simulink model "DFADAS2_SenFus_v1_201204RC_training_210115"  (R2018b)
settings: Solver=FixedStepDiscrete  StartTime=0.0  StopTime=inf  FixedStep=0.002  RelTol=1e-3  EnableMultiTasking=on
PreLoadFcn:
  | RTWConfigurationCB('preloadfcn', bdroot);
libraries: canmsglib x108, simulink x48, canfdmsglib x12
(part 8 of 28)

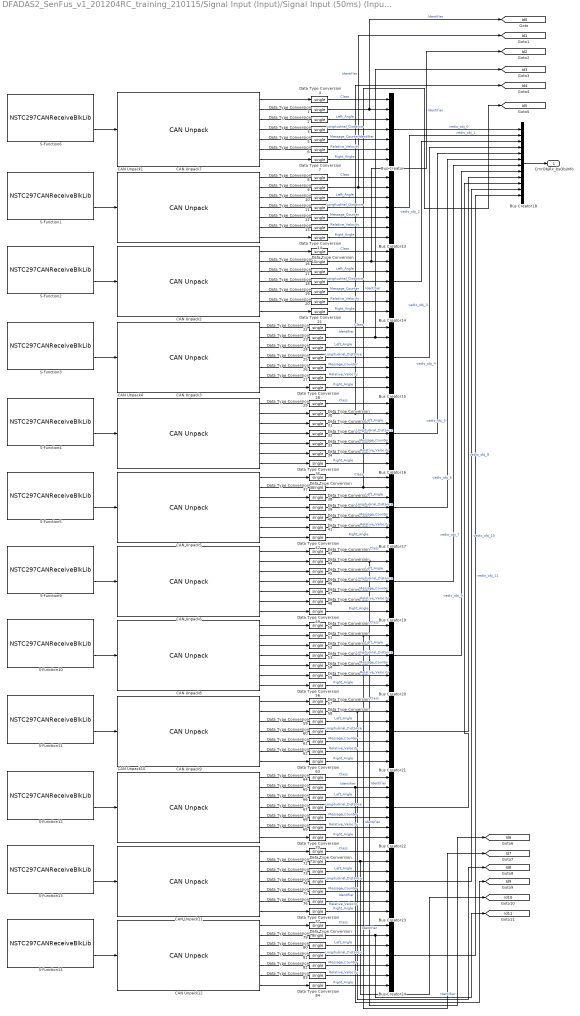
== system DFADAS2_SenFus_v1_201204RC_training_210115/Signal Input (Input)/Signal Input (50ms) (Input50)/Cmr/Camera Objects Information (CmrObjInfo) ==
  Bus Creator{,13..17,19..24} (12 alike) : BusCreator  Inputs=7
  Bus Creator18 : BusCreator  Inputs=12
  CAN Unpack1 : canmsglib/CAN Unpack  CANdbFile=F:\V_control\ADAS ECU-Sensor CAN_V2_20190314(1).dbc  MsgList=Video_Object_1_A  MsgName=Video_Object_1_A  MsgIDType=Standard (11-bit identifier)  MsgIdentifier=1796  MsgLength=8  SignalInfo=Class_704$56$3$2$2$1$0$1$0$0$7$#Identifier_704$1$7$2$2$1$0$1$0$0$127$#Left_Angle_704$41$13$2$1$1$0$2.000000e-04$0$-8.192000e-01$8.190000e-01$#Longitudinal_Distance_704$20$12$2$2$1$0$5.000000e-02$0$0$2.047500e+02$#Message_Counter_704$38$2$2$2$1$0$1$0$0$3$#Relative_Velocity_704$24$12$2$1$1$0$5.000000e-02$0$-1.024000e+02$1.023500e+02$#Right_Angle_704$59$13$2$1$1$0$2.000000e-04$0$-8.192000e-01$8.190000e-01$#  NSignals=7  IDPort=off  TimestampPort=off  ErrorPort=off  RemotePort=off  LengthPort=off  StatusPort=off  StartBits=str2num('[int32(56);int32(1);int32(41);int32(20);int32(38);int32(24);int32(59)]')  SignalSizes=str2num('[int32(3);int32(7);int32(13);int32(12);int32(2);int32(12);int32(13)]')  ByteOrders=str2num('[int32(2);int32(2);int32(2);int32(2);int32(2);int32(2);int32(2)]')  DataTypes=str2num('[int32(2);int32(2);int32(1);int32(2);int32(2);int32(1);int32(1)]')  MultiplexTypes=str2num('[int32(1);int32(1);int32(1);int32(1);int32(1);int32(1);int32(1)]')  MultiplexValues=str2num('[double(0);double(0);double(0);double(0);double(0);double(0);double(0)]')  Factors=str2num('[double(1);double(1);double(2.000000e-04);double(5.000000e-02);double(1);double(5.000000e-02);double(2.000000e-04)]')  Offsets=str2num('[double(0);double(0);double(0);double(0);double(0);double(0);double(0)]')  Minimums=str2num('[double(0);double(0);double(-8.192000e-01);double(0);double(0);double(-1.024000e+02);double(-8.192000e-01)]')  Maximums=str2num('[double(7);double(127);double(8.190000e-01);double(2.047500e+02);double(3);double(1.023500e+02);double(8.190000e-01)]')  ApplyMinMax=off
      settings: SourceProductName=Simulink Real-Time  SourceProductBaseCode=XP  DataFormat=CANdb specified signals
  CAN Unpack10 : canmsglib/CAN Unpack  CANdbFile=F:\V_control\ADAS ECU-Sensor CAN_V2_20190314(1).dbc  MsgList=Video_Object_9_A  MsgName=Video_Object_9_A  MsgIDType=Standard (11-bit identifier)  MsgIdentifier=1828  MsgLength=8  SignalInfo=Class_724$56$3$2$2$1$0$1$0$0$7$#Identifier_724$1$7$2$2$1$0$1$0$0$127$#Left_Angle_724$41$13$2$1$1$0$2.000000e-04$0$-8.192000e-01$8.190000e-01$#Longitudinal_Distance_724$20$12$2$2$1$0$5.000000e-02$0$0$2.047500e+02$#Message_Counter_724$38$2$2$2$1$0$1$0$0$3$#Relative_Velocity_724$24$12$2$1$1$0$5.000000e-02$0$-1.024000e+02$1.023500e+02$#Right_Angle_724$59$13$2$1$1$0$2.000000e-04$0$-8.192000e-01$8.190000e-01$#  NSignals=7  IDPort=off  TimestampPort=off  ErrorPort=off  RemotePort=off  LengthPort=off  StatusPort=off  StartBits=str2num('[int32(56);int32(1);int32(41);int32(20);int32(38);int32(24);int32(59)]')  SignalSizes=str2num('[int32(3);int32(7);int32(13);int32(12);int32(2);int32(12);int32(13)]')  ByteOrders=str2num('[int32(2);int32(2);int32(2);int32(2);int32(2);int32(2);int32(2)]')  DataTypes=str2num('[int32(2);int32(2);int32(1);int32(2);int32(2);int32(1);int32(1)]')  MultiplexTypes=str2num('[int32(1);int32(1);int32(1);int32(1);int32(1);int32(1);int32(1)]')  MultiplexValues=str2num('[double(0);double(0);double(0);double(0);double(0);double(0);double(0)]')  Factors=str2num('[double(1);double(1);double(2.000000e-04);double(5.000000e-02);double(1);double(5.000000e-02);double(2.000000e-04)]')  Offsets=str2num('[double(0);double(0);double(0);double(0);double(0);double(0);double(0)]')  Minimums=str2num('[double(0);double(0);double(-8.192000e-01);double(0);double(0);double(-1.024000e+02);double(-8.192000e-01)]')  Maximums=str2num('[double(7);double(127);double(8.190000e-01);double(2.047500e+02);double(3);double(1.023500e+02);double(8.190000e-01)]')  ApplyMinMax=off
      settings: SourceProductName=Simulink Real-Time  SourceProductBaseCode=XP  DataFormat=CANdb specified signals
  CAN Unpack11 : canmsglib/CAN Unpack  CANdbFile=F:\V_control\ADAS ECU-Sensor CAN_V2_20190314(1).dbc  MsgList=Video_Object_10_A  MsgName=Video_Object_10_A  MsgIDType=Standard (11-bit identifier)  MsgIdentifier=1832  MsgLength=8  SignalInfo=Class_728$56$3$2$2$1$0$1$0$0$7$#Identifier_728$1$7$2$2$1$0$1$0$0$127$#Left_Angle_728$41$13$2$1$1$0$2.000000e-04$0$-8.192000e-01$8.190000e-01$#Longitudinal_Distance_728$20$12$2$2$1$0$5.000000e-02$0$0$2.047500e+02$#Message_Counter_728$38$2$2$2$1$0$1$0$0$3$#Relative_Velocity_728$24$12$2$1$1$0$5.000000e-02$0$-1.024000e+02$1.023500e+02$#Right_Angle_728$59$13$2$1$1$0$2.000000e-04$0$-8.192000e-01$8.190000e-01$#  NSignals=7  IDPort=off  TimestampPort=off  ErrorPort=off  RemotePort=off  LengthPort=off  StatusPort=off  StartBits=str2num('[int32(56);int32(1);int32(41);int32(20);int32(38);int32(24);int32(59)]')  SignalSizes=str2num('[int32(3);int32(7);int32(13);int32(12);int32(2);int32(12);int32(13)]')  ByteOrders=str2num('[int32(2);int32(2);int32(2);int32(2);int32(2);int32(2);int32(2)]')  DataTypes=str2num('[int32(2);int32(2);int32(1);int32(2);int32(2);int32(1);int32(1)]')  MultiplexTypes=str2num('[int32(1);int32(1);int32(1);int32(1);int32(1);int32(1);int32(1)]')  MultiplexValues=str2num('[double(0);double(0);double(0);double(0);double(0);double(0);double(0)]')  Factors=str2num('[double(1);double(1);double(2.000000e-04);double(5.000000e-02);double(1);double(5.000000e-02);double(2.000000e-04)]')  Offsets=str2num('[double(0);double(0);double(0);double(0);double(0);double(0);double(0)]')  Minimums=str2num('[double(0);double(0);double(-8.192000e-01);double(0);double(0);double(-1.024000e+02);double(-8.192000e-01)]')  Maximums=str2num('[double(7);double(127);double(8.190000e-01);double(2.047500e+02);double(3);double(1.023500e+02);double(8.190000e-01)]')  ApplyMinMax=off
      settings: SourceProductName=Simulink Real-Time  SourceProductBaseCode=XP  DataFormat=CANdb specified signals
  CAN Unpack12 : canmsglib/CAN Unpack  CANdbFile=F:\V_control\ADAS ECU-Sensor CAN_V2_20190314(1).dbc  MsgList=Video_Object_11_A  MsgName=Video_Object_11_A  MsgIDType=Standard (11-bit identifier)  MsgIdentifier=1836  MsgLength=8  SignalInfo=Class_72C$56$3$2$2$1$0$1$0$0$7$#Identifier_72C$1$7$2$2$1$0$1$0$0$127$#Left_Angle_72C$41$13$2$1$1$0$2.000000e-04$0$-8.192000e-01$8.190000e-01$#Longitudinal_Distance_72C$20$12$2$2$1$0$5.000000e-02$0$0$2.047500e+02$#Message_Counter_72C$38$2$2$2$1$0$1$0$0$3$#Relative_Velocity_72C$24$12$2$1$1$0$5.000000e-02$0$-1.024000e+02$1.023500e+02$#Right_Angle_72C$59$13$2$1$1$0$2.000000e-04$0$-8.192000e-01$8.190000e-01$#  NSignals=7  IDPort=off  TimestampPort=off  ErrorPort=off  RemotePort=off  LengthPort=off  StatusPort=off  StartBits=str2num('[int32(56);int32(1);int32(41);int32(20);int32(38);int32(24);int32(59)]')  SignalSizes=str2num('[int32(3);int32(7);int32(13);int32(12);int32(2);int32(12);int32(13)]')  ByteOrders=str2num('[int32(2);int32(2);int32(2);int32(2);int32(2);int32(2);int32(2)]')  DataTypes=str2num('[int32(2);int32(2);int32(1);int32(2);int32(2);int32(1);int32(1)]')  MultiplexTypes=str2num('[int32(1);int32(1);int32(1);int32(1);int32(1);int32(1);int32(1)]')  MultiplexValues=str2num('[double(0);double(0);double(0);double(0);double(0);double(0);double(0)]')  Factors=str2num('[double(1);double(1);double(2.000000e-04);double(5.000000e-02);double(1);double(5.000000e-02);double(2.000000e-04)]')  Offsets=str2num('[double(0);double(0);double(0);double(0);double(0);double(0);double(0)]')  Minimums=str2num('[double(0);double(0);double(-8.192000e-01);double(0);double(0);double(-1.024000e+02);double(-8.192000e-01)]')  Maximums=str2num('[double(7);double(127);double(8.190000e-01);double(2.047500e+02);double(3);double(1.023500e+02);double(8.190000e-01)]')  ApplyMinMax=off
      settings: SourceProductName=Simulink Real-Time  SourceProductBaseCode=XP  DataFormat=CANdb specified signals
  CAN Unpack2 : canmsglib/CAN Unpack  CANdbFile=F:\V_control\ADAS ECU-Sensor CAN_V2_20190314(1).dbc  MsgList=Video_Object_2_A  MsgName=Video_Object_2_A  MsgIDType=Standard (11-bit identifier)  MsgIdentifier=1800  MsgLength=8  SignalInfo=Class_708$56$3$2$2$1$0$1$0$0$7$#Identifier_708$1$7$2$2$1$0$1$0$0$127$#Left_Angle_708$41$13$2$1$1$0$2.000000e-04$0$-8.192000e-01$8.190000e-01$#Longitudinal_Distance_708$20$12$2$2$1$0$5.000000e-02$0$0$2.047500e+02$#Message_Counter_708$38$2$2$2$1$0$1$0$0$3$#Relative_Velocity_708$24$12$2$1$1$0$5.000000e-02$0$-1.024000e+02$1.023500e+02$#Right_Angle_708$59$13$2$1$1$0$2.000000e-04$0$-8.192000e-01$8.190000e-01$#  NSignals=7  IDPort=off  TimestampPort=off  ErrorPort=off  RemotePort=off  LengthPort=off  StatusPort=off  StartBits=str2num('[int32(56);int32(1);int32(41);int32(20);int32(38);int32(24);int32(59)]')  SignalSizes=str2num('[int32(3);int32(7);int32(13);int32(12);int32(2);int32(12);int32(13)]')  ByteOrders=str2num('[int32(2);int32(2);int32(2);int32(2);int32(2);int32(2);int32(2)]')  DataTypes=str2num('[int32(2);int32(2);int32(1);int32(2);int32(2);int32(1);int32(1)]')  MultiplexTypes=str2num('[int32(1);int32(1);int32(1);int32(1);int32(1);int32(1);int32(1)]')  MultiplexValues=str2num('[double(0);double(0);double(0);double(0);double(0);double(0);double(0)]')  Factors=str2num('[double(1);double(1);double(2.000000e-04);double(5.000000e-02);double(1);double(5.000000e-02);double(2.000000e-04)]')  Offsets=str2num('[double(0);double(0);double(0);double(0);double(0);double(0);double(0)]')  Minimums=str2num('[double(0);double(0);double(-8.192000e-01);double(0);double(0);double(-1.024000e+02);double(-8.192000e-01)]')  Maximums=str2num('[double(7);double(127);double(8.190000e-01);double(2.047500e+02);double(3);double(1.023500e+02);double(8.190000e-01)]')  ApplyMinMax=off
      settings: SourceProductName=Simulink Real-Time  SourceProductBaseCode=XP  DataFormat=CANdb specified signals
  CAN Unpack3 : canmsglib/CAN Unpack  CANdbFile=F:\V_control\ADAS ECU-Sensor CAN_V2_20190314(1).dbc  MsgList=Video_Object_3_A  MsgName=Video_Object_3_A  MsgIDType=Standard (11-bit identifier)  MsgIdentifier=1804  MsgLength=8  SignalInfo=Class_70C$56$3$2$2$1$0$1$0$0$7$#Identifier_70C$1$7$2$2$1$0$1$0$0$127$#Left_Angle_70C$41$13$2$1$1$0$2.000000e-04$0$-8.192000e-01$8.190000e-01$#Longitudinal_Distance_70C$20$12$2$2$1$0$5.000000e-02$0$0$2.047500e+02$#Message_Counter_70C$38$2$2$2$1$0$1$0$0$3$#Relative_Velocity_70C$24$12$2$1$1$0$5.000000e-02$0$-1.024000e+02$1.023500e+02$#Right_Angle_70C$59$13$2$1$1$0$2.000000e-04$0$-8.192000e-01$8.190000e-01$#  NSignals=7  IDPort=off  TimestampPort=off  ErrorPort=off  RemotePort=off  LengthPort=off  StatusPort=off  StartBits=str2num('[int32(56);int32(1);int32(41);int32(20);int32(38);int32(24);int32(59)]')  SignalSizes=str2num('[int32(3);int32(7);int32(13);int32(12);int32(2);int32(12);int32(13)]')  ByteOrders=str2num('[int32(2);int32(2);int32(2);int32(2);int32(2);int32(2);int32(2)]')  DataTypes=str2num('[int32(2);int32(2);int32(1);int32(2);int32(2);int32(1);int32(1)]')  MultiplexTypes=str2num('[int32(1);int32(1);int32(1);int32(1);int32(1);int32(1);int32(1)]')  MultiplexValues=str2num('[double(0);double(0);double(0);double(0);double(0);double(0);double(0)]')  Factors=str2num('[double(1);double(1);double(2.000000e-04);double(5.000000e-02);double(1);double(5.000000e-02);double(2.000000e-04)]')  Offsets=str2num('[double(0);double(0);double(0);double(0);double(0);double(0);double(0)]')  Minimums=str2num('[double(0);double(0);double(-8.192000e-01);double(0);double(0);double(-1.024000e+02);double(-8.192000e-01)]')  Maximums=str2num('[double(7);double(127);double(8.190000e-01);double(2.047500e+02);double(3);double(1.023500e+02);double(8.190000e-01)]')  ApplyMinMax=off
      settings: SourceProductName=Simulink Real-Time  SourceProductBaseCode=XP  DataFormat=CANdb specified signals
  CAN Unpack4 : canmsglib/CAN Unpack  CANdbFile=F:\V_control\ADAS ECU-Sensor CAN_V2_20190314(1).dbc  MsgList=Video_Object_4_A  MsgName=Video_Object_4_A  MsgIDType=Standard (11-bit identifier)  MsgIdentifier=1808  MsgLength=8  SignalInfo=Class_710$56$3$2$2$1$0$1$0$0$7$#Identifier_710$1$7$2$2$1$0$1$0$0$127$#Left_Angle_710$41$13$2$1$1$0$2.000000e-04$0$-8.192000e-01$8.190000e-01$#Longitudinal_Distance_710$20$12$2$2$1$0$5.000000e-02$0$0$2.047500e+02$#Message_Counter_710$38$2$2$2$1$0$1$0$0$3$#Relative_Velocity_710$24$12$2$1$1$0$5.000000e-02$0$-1.024000e+02$1.023500e+02$#Right_Angle_710$59$13$2$1$1$0$2.000000e-04$0$-8.192000e-01$8.190000e-01$#  NSignals=7  IDPort=off  TimestampPort=off  ErrorPort=off  RemotePort=off  LengthPort=off  StatusPort=off  StartBits=str2num('[int32(56);int32(1);int32(41);int32(20);int32(38);int32(24);int32(59)]')  SignalSizes=str2num('[int32(3);int32(7);int32(13);int32(12);int32(2);int32(12);int32(13)]')  ByteOrders=str2num('[int32(2);int32(2);int32(2);int32(2);int32(2);int32(2);int32(2)]')  DataTypes=str2num('[int32(2);int32(2);int32(1);int32(2);int32(2);int32(1);int32(1)]')  MultiplexTypes=str2num('[int32(1);int32(1);int32(1);int32(1);int32(1);int32(1);int32(1)]')  MultiplexValues=str2num('[double(0);double(0);double(0);double(0);double(0);double(0);double(0)]')  Factors=str2num('[double(1);double(1);double(2.000000e-04);double(5.000000e-02);double(1);double(5.000000e-02);double(2.000000e-04)]')  Offsets=str2num('[double(0);double(0);double(0);double(0);double(0);double(0);double(0)]')  Minimums=str2num('[double(0);double(0);double(-8.192000e-01);double(0);double(0);double(-1.024000e+02);double(-8.192000e-01)]')  Maximums=str2num('[double(7);double(127);double(8.190000e-01);double(2.047500e+02);double(3);double(1.023500e+02);double(8.190000e-01)]')  ApplyMinMax=off
      settings: SourceProductName=Simulink Real-Time  SourceProductBaseCode=XP  DataFormat=CANdb specified signals
  CAN Unpack5 : canmsglib/CAN Unpack  CANdbFile=F:\V_control\ADAS ECU-Sensor CAN_V2_20190314(1).dbc  MsgList=Video_Object_5_A  MsgName=Video_Object_5_A  MsgIDType=Standard (11-bit identifier)  MsgIdentifier=1812  MsgLength=8  SignalInfo=Class_714$56$3$2$2$1$0$1$0$0$7$#Identifier_714$1$7$2$2$1$0$1$0$0$127$#Left_Angle_714$41$13$2$1$1$0$2.000000e-04$0$-8.192000e-01$8.190000e-01$#Longitudinal_Distance_714$20$12$2$2$1$0$5.000000e-02$0$0$2.047500e+02$#Message_Counter_714$38$2$2$2$1$0$1$0$0$3$#Relative_Velocity_714$24$12$2$1$1$0$5.000000e-02$0$-1.024000e+02$1.023500e+02$#Right_Angle_714$59$13$2$1$1$0$2.000000e-04$0$-8.192000e-01$8.190000e-01$#  NSignals=7  IDPort=off  TimestampPort=off  ErrorPort=off  RemotePort=off  LengthPort=off  StatusPort=off  StartBits=str2num('[int32(56);int32(1);int32(41);int32(20);int32(38);int32(24);int32(59)]')  SignalSizes=str2num('[int32(3);int32(7);int32(13);int32(12);int32(2);int32(12);int32(13)]')  ByteOrders=str2num('[int32(2);int32(2);int32(2);int32(2);int32(2);int32(2);int32(2)]')  DataTypes=str2num('[int32(2);int32(2);int32(1);int32(2);int32(2);int32(1);int32(1)]')  MultiplexTypes=str2num('[int32(1);int32(1);int32(1);int32(1);int32(1);int32(1);int32(1)]')  MultiplexValues=str2num('[double(0);double(0);double(0);double(0);double(0);double(0);double(0)]')  Factors=str2num('[double(1);double(1);double(2.000000e-04);double(5.000000e-02);double(1);double(5.000000e-02);double(2.000000e-04)]')  Offsets=str2num('[double(0);double(0);double(0);double(0);double(0);double(0);double(0)]')  Minimums=str2num('[double(0);double(0);double(-8.192000e-01);double(0);double(0);double(-1.024000e+02);double(-8.192000e-01)]')  Maximums=str2num('[double(7);double(127);double(8.190000e-01);double(2.047500e+02);double(3);double(1.023500e+02);double(8.190000e-01)]')  ApplyMinMax=off
      settings: SourceProductName=Simulink Real-Time  SourceProductBaseCode=XP  DataFormat=CANdb specified signals
  CAN Unpack6 : canmsglib/CAN Unpack  CANdbFile=F:\V_control\ADAS ECU-Sensor CAN_V2_20190314(1).dbc  MsgList=Video_Object_6_A  MsgName=Video_Object_6_A  MsgIDType=Standard (11-bit identifier)  MsgIdentifier=1816  MsgLength=8  SignalInfo=Class_718$56$3$2$2$1$0$1$0$0$7$#Identifier_718$1$7$2$2$1$0$1$0$0$127$#Left_Angle_718$41$13$2$1$1$0$2.000000e-04$0$-8.192000e-01$8.190000e-01$#Longitudinal_Distance_718$20$12$2$2$1$0$5.000000e-02$0$0$2.047500e+02$#Message_Counter_718$38$2$2$2$1$0$1$0$0$3$#Relative_Velocity_718$24$12$2$1$1$0$5.000000e-02$0$-1.024000e+02$1.023500e+02$#Right_Angle_718$59$13$2$1$1$0$2.000000e-04$0$-8.192000e-01$8.190000e-01$#  NSignals=7  IDPort=off  TimestampPort=off  ErrorPort=off  RemotePort=off  LengthPort=off  StatusPort=off  StartBits=str2num('[int32(56);int32(1);int32(41);int32(20);int32(38);int32(24);int32(59)]')  SignalSizes=str2num('[int32(3);int32(7);int32(13);int32(12);int32(2);int32(12);int32(13)]')  ByteOrders=str2num('[int32(2);int32(2);int32(2);int32(2);int32(2);int32(2);int32(2)]')  DataTypes=str2num('[int32(2);int32(2);int32(1);int32(2);int32(2);int32(1);int32(1)]')  MultiplexTypes=str2num('[int32(1);int32(1);int32(1);int32(1);int32(1);int32(1);int32(1)]')  MultiplexValues=str2num('[double(0);double(0);double(0);double(0);double(0);double(0);double(0)]')  Factors=str2num('[double(1);double(1);double(2.000000e-04);double(5.000000e-02);double(1);double(5.000000e-02);double(2.000000e-04)]')  Offsets=str2num('[double(0);double(0);double(0);double(0);double(0);double(0);double(0)]')  Minimums=str2num('[double(0);double(0);double(-8.192000e-01);double(0);double(0);double(-1.024000e+02);double(-8.192000e-01)]')  Maximums=str2num('[double(7);double(127);double(8.190000e-01);double(2.047500e+02);double(3);double(1.023500e+02);double(8.190000e-01)]')  ApplyMinMax=off
      settings: SourceProductName=Simulink Real-Time  SourceProductBaseCode=XP  DataFormat=CANdb specified signals
  CAN Unpack7 : canmsglib/CAN Unpack  CANdbFile=F:\V_control\ADAS ECU-Sensor CAN_V2_20190314(1).dbc  MsgList=Video_Object_0_A  MsgName=Video_Object_0_A  MsgIDType=Standard (11-bit identifier)  MsgIdentifier=1792  MsgLength=8  SignalInfo=Class_700$56$3$2$2$1$0$1$0$0$7$#Identifier_700$1$7$2$2$1$0$1$0$0$127$#Left_Angle_700$41$13$2$1$1$0$2.000000e-04$0$-8.192000e-01$8.190000e-01$#Longitudinal_Distance_700$20$12$2$2$1$0$5.000000e-02$0$0$2.047500e+02$#Message_Counter_700$38$2$2$2$1$0$1$0$0$3$#Relative_Velocity_700$24$12$2$1$1$0$5.000000e-02$0$-1.024000e+02$1.023500e+02$#Right_Angle_700$59$13$2$1$1$0$2.000000e-04$0$-8.192000e-01$8.190000e-01$#  NSignals=7  IDPort=off  TimestampPort=off  ErrorPort=off  RemotePort=off  LengthPort=off  StatusPort=off  StartBits=str2num('[int32(56);int32(1);int32(41);int32(20);int32(38);int32(24);int32(59)]')  SignalSizes=str2num('[int32(3);int32(7);int32(13);int32(12);int32(2);int32(12);int32(13)]')  ByteOrders=str2num('[int32(2);int32(2);int32(2);int32(2);int32(2);int32(2);int32(2)]')  DataTypes=str2num('[int32(2);int32(2);int32(1);int32(2);int32(2);int32(1);int32(1)]')  MultiplexTypes=str2num('[int32(1);int32(1);int32(1);int32(1);int32(1);int32(1);int32(1)]')  MultiplexValues=str2num('[double(0);double(0);double(0);double(0);double(0);double(0);double(0)]')  Factors=str2num('[double(1);double(1);double(2.000000e-04);double(5.000000e-02);double(1);double(5.000000e-02);double(2.000000e-04)]')  Offsets=str2num('[double(0);double(0);double(0);double(0);double(0);double(0);double(0)]')  Minimums=str2num('[double(0);double(0);double(-8.192000e-01);double(0);double(0);double(-1.024000e+02);double(-8.192000e-01)]')  Maximums=str2num('[double(7);double(127);double(8.190000e-01);double(2.047500e+02);double(3);double(1.023500e+02);double(8.190000e-01)]')  ApplyMinMax=off
      settings: SourceProductName=Simulink Real-Time  SourceProductBaseCode=XP  DataFormat=CANdb specified signals
  CAN Unpack8 : canmsglib/CAN Unpack  CANdbFile=F:\V_control\ADAS ECU-Sensor CAN_V2_20190314(1).dbc  MsgList=Video_Object_7_A  MsgName=Video_Object_7_A  MsgIDType=Standard (11-bit identifier)  MsgIdentifier=1820  MsgLength=8  SignalInfo=Class_71C$56$3$2$2$1$0$1$0$0$7$#Identifier_71C$1$7$2$2$1$0$1$0$0$127$#Left_Angle_71C$41$13$2$1$1$0$2.000000e-04$0$-8.192000e-01$8.190000e-01$#Longitudinal_Distance_71C$20$12$2$2$1$0$5.000000e-02$0$0$2.047500e+02$#Message_Counter_71C$38$2$2$2$1$0$1$0$0$3$#Relative_Velocity_71C$24$12$2$1$1$0$5.000000e-02$0$-1.024000e+02$1.023500e+02$#Right_Angle_71C$59$13$2$1$1$0$2.000000e-04$0$-8.192000e-01$8.190000e-01$#  NSignals=7  IDPort=off  TimestampPort=off  ErrorPort=off  RemotePort=off  LengthPort=off  StatusPort=off  StartBits=str2num('[int32(56);int32(1);int32(41);int32(20);int32(38);int32(24);int32(59)]')  SignalSizes=str2num('[int32(3);int32(7);int32(13);int32(12);int32(2);int32(12);int32(13)]')  ByteOrders=str2num('[int32(2);int32(2);int32(2);int32(2);int32(2);int32(2);int32(2)]')  DataTypes=str2num('[int32(2);int32(2);int32(1);int32(2);int32(2);int32(1);int32(1)]')  MultiplexTypes=str2num('[int32(1);int32(1);int32(1);int32(1);int32(1);int32(1);int32(1)]')  MultiplexValues=str2num('[double(0);double(0);double(0);double(0);double(0);double(0);double(0)]')  Factors=str2num('[double(1);double(1);double(2.000000e-04);double(5.000000e-02);double(1);double(5.000000e-02);double(2.000000e-04)]')  Offsets=str2num('[double(0);double(0);double(0);double(0);double(0);double(0);double(0)]')  Minimums=str2num('[double(0);double(0);double(-8.192000e-01);double(0);double(0);double(-1.024000e+02);double(-8.192000e-01)]')  Maximums=str2num('[double(7);double(127);double(8.190000e-01);double(2.047500e+02);double(3);double(1.023500e+02);double(8.190000e-01)]')  ApplyMinMax=off
      settings: SourceProductName=Simulink Real-Time  SourceProductBaseCode=XP  DataFormat=CANdb specified signals
  CAN Unpack9 : canmsglib/CAN Unpack  CANdbFile=F:\V_control\ADAS ECU-Sensor CAN_V2_20190314(1).dbc  MsgList=Video_Object_8_A  MsgName=Video_Object_8_A  MsgIDType=Standard (11-bit identifier)  MsgIdentifier=1824  MsgLength=8  SignalInfo=Class_720$56$3$2$2$1$0$1$0$0$7$#Identifier_720$1$7$2$2$1$0$1$0$0$127$#Left_Angle_720$41$13$2$1$1$0$2.000000e-04$0$-8.192000e-01$8.190000e-01$#Longitudinal_Distance_720$20$12$2$2$1$0$5.000000e-02$0$0$2.047500e+02$#Message_Counter_720$38$2$2$2$1$0$1$0$0$3$#Relative_Velocity_720$24$12$2$1$1$0$5.000000e-02$0$-1.024000e+02$1.023500e+02$#Right_Angle_720$59$13$2$1$1$0$2.000000e-04$0$-8.192000e-01$8.190000e-01$#  NSignals=7  IDPort=off  TimestampPort=off  ErrorPort=off  RemotePort=off  LengthPort=off  StatusPort=off  StartBits=str2num('[int32(56);int32(1);int32(41);int32(20);int32(38);int32(24);int32(59)]')  SignalSizes=str2num('[int32(3);int32(7);int32(13);int32(12);int32(2);int32(12);int32(13)]')  ByteOrders=str2num('[int32(2);int32(2);int32(2);int32(2);int32(2);int32(2);int32(2)]')  DataTypes=str2num('[int32(2);int32(2);int32(1);int32(2);int32(2);int32(1);int32(1)]')  MultiplexTypes=str2num('[int32(1);int32(1);int32(1);int32(1);int32(1);int32(1);int32(1)]')  MultiplexValues=str2num('[double(0);double(0);double(0);double(0);double(0);double(0);double(0)]')  Factors=str2num('[double(1);double(1);double(2.000000e-04);double(5.000000e-02);double(1);double(5.000000e-02);double(2.000000e-04)]')  Offsets=str2num('[double(0);double(0);double(0);double(0);double(0);double(0);double(0)]')  Minimums=str2num('[double(0);double(0);double(-8.192000e-01);double(0);double(0);double(-1.024000e+02);double(-8.192000e-01)]')  Maximums=str2num('[double(7);double(127);double(8.190000e-01);double(2.047500e+02);double(3);double(1.023500e+02);double(8.190000e-01)]')  ApplyMinMax=off
      settings: SourceProductName=Simulink Real-Time  SourceProductBaseCode=XP  DataFormat=CANdb specified signals
  Data Type Conversion{1..84} (84 alike) : DataTypeConversion  OutDataTypeStr=single
  S-Function1 : S-Function  FunctionName=NSTC297CANReceiveBlkLib  Parameters=|  SFunctionDeploymentMode=off  EnableBusSupport=off  mask(NSTC297 CAN Receive){Ns_DeviceID=ADAS Control Unit Gen2, Ns_ChannelNum=5, Ns_FrameID=1796, Ns_IsVirtualFrame=off, Ns_RoleInVirtualFrame=Header Frame, Ns_HeaderFrameID=0, Ns_VirtualFrameStatusFlg=off, Ns_IncompleteFrameCntFlg=off, Ns_OverflowCntFlg=off, Ns_FrameBufferSize=1, Ns_SampleTime=0.05}
      | uint16(Ns_DeviceID),
      | uint16(Ns_ChannelNum),
      | uint32(Ns_FrameID),
      | uint8(Ns_IsVirtualFrame),
      | uint16(Ns_RoleInVirtualFrame),
      | uint32(Ns_HeaderFrameID),
      | uint8(Ns_VirtualFrameStatusFlg),
      | uint8(Ns_IncompleteFrameCntFlg),
      | uint8(Ns_OverflowCntFlg),
      | uint16(Ns_FrameBufferSize),
      | double(Ns_SampleTime)
      mask prompts: Ns_DeviceID "Device:"; Ns_ChannelNum "Channel number:"; Ns_FrameID "Frame ID:"; Ns_IsVirtualFrame "Belong to a virtual frame"; Ns_RoleInVirtualFrame "Position in virtual frame:"; Ns_HeaderFrameID "Header frame ID:"; Ns_VirtualFrameStatusFlg "Current virtural frame status output"; Ns_IncompleteFrameCntFlg "Incomplete virtual frame count output"; Ns_OverflowCntFlg "Overflow count output"; Ns_FrameBufferSize "Frame buffer size:"; Ns_SampleTime "Sample time:"
      mask init:
      | NSTC297CANReceive_callback('portlabels');
      mask TypeOptions Ns_DeviceID: General Control Unit Gen2 | ADAS Control Unit Gen2
      mask TypeOptions Ns_ChannelNum: 0 | 1 | 2 | 3 | 4 | 5
      mask Callback Ns_IsVirtualFrame: NSTC297CANReceive_callback('Belong to a virtual frame');
      mask TypeOptions Ns_RoleInVirtualFrame: Header Frame | Data Frame | Trailer Frame
      mask Callback Ns_RoleInVirtualFrame: NSTC297CANReceive_callback('Position in virtual frame');
      mask Display: color('blue');text(0.02,0.9,'NovSteeds TC297','horizontalAlignment','left');color('blue');text(0.5,0.7,'CAN Receive','horizontalAlignment','center');color('black');text(0.5,0.6,'Channel: 5','horizontalAlignment','center');text(0.5,0.5,'ID: 1796','horizontalAlignment','center');text(0.5,0.4,'Virtual Frame: No','horizontalAlignment','center');port_label('output',1, 'RemainderCnt');port_label('output',2, 'Msg');
  S-Function10 : S-Function  FunctionName=NSTC297CANReceiveBlkLib  Parameters=|  SFunctionDeploymentMode=off  EnableBusSupport=off  mask(NSTC297 CAN Receive){Ns_DeviceID=ADAS Control Unit Gen2, Ns_ChannelNum=5, Ns_FrameID=1820, Ns_IsVirtualFrame=off, Ns_RoleInVirtualFrame=Header Frame, Ns_HeaderFrameID=0, Ns_VirtualFrameStatusFlg=off, Ns_IncompleteFrameCntFlg=off, Ns_OverflowCntFlg=off, Ns_FrameBufferSize=1, Ns_SampleTime=0.05}
      | uint16(Ns_DeviceID),
      | uint16(Ns_ChannelNum),
      | uint32(Ns_FrameID),
      | uint8(Ns_IsVirtualFrame),
      | uint16(Ns_RoleInVirtualFrame),
      | uint32(Ns_HeaderFrameID),
      | uint8(Ns_VirtualFrameStatusFlg),
      | uint8(Ns_IncompleteFrameCntFlg),
      | uint8(Ns_OverflowCntFlg),
      | uint16(Ns_FrameBufferSize),
      | double(Ns_SampleTime)
      mask prompts: Ns_DeviceID "Device:"; Ns_ChannelNum "Channel number:"; Ns_FrameID "Frame ID:"; Ns_IsVirtualFrame "Belong to a virtual frame"; Ns_RoleInVirtualFrame "Position in virtual frame:"; Ns_HeaderFrameID "Header frame ID:"; Ns_VirtualFrameStatusFlg "Current virtural frame status output"; Ns_IncompleteFrameCntFlg "Incomplete virtual frame count output"; Ns_OverflowCntFlg "Overflow count output"; Ns_FrameBufferSize "Frame buffer size:"; Ns_SampleTime "Sample time:"
      mask init:
      | NSTC297CANReceive_callback('portlabels');
      mask TypeOptions Ns_DeviceID: General Control Unit Gen2 | ADAS Control Unit Gen2
      mask TypeOptions Ns_ChannelNum: 0 | 1 | 2 | 3 | 4 | 5
      mask Callback Ns_IsVirtualFrame: NSTC297CANReceive_callback('Belong to a virtual frame');
      mask TypeOptions Ns_RoleInVirtualFrame: Header Frame | Data Frame | Trailer Frame
      mask Callback Ns_RoleInVirtualFrame: NSTC297CANReceive_callback('Position in virtual frame');
      mask Display: color('blue');text(0.02,0.9,'NovSteeds TC297','horizontalAlignment','left');color('blue');text(0.5,0.7,'CAN Receive','horizontalAlignment','center');color('black');text(0.5,0.6,'Channel: 5','horizontalAlignment','center');text(0.5,0.5,'ID: 1820','horizontalAlignment','center');text(0.5,0.4,'Virtual Frame: No','horizontalAlignment','center');port_label('output',1, 'RemainderCnt');port_label('output',2, 'Msg');
  S-Function11 : S-Function  FunctionName=NSTC297CANReceiveBlkLib  Parameters=|  SFunctionDeploymentMode=off  EnableBusSupport=off  mask(NSTC297 CAN Receive){Ns_DeviceID=ADAS Control Unit Gen2, Ns_ChannelNum=5, Ns_FrameID=1824, Ns_IsVirtualFrame=off, Ns_RoleInVirtualFrame=Header Frame, Ns_HeaderFrameID=0, Ns_VirtualFrameStatusFlg=off, Ns_IncompleteFrameCntFlg=off, Ns_OverflowCntFlg=off, Ns_FrameBufferSize=1, Ns_SampleTime=0.05}
      | uint16(Ns_DeviceID),
      | uint16(Ns_ChannelNum),
      | uint32(Ns_FrameID),
      | uint8(Ns_IsVirtualFrame),
      | uint16(Ns_RoleInVirtualFrame),
      | uint32(Ns_HeaderFrameID),
      | uint8(Ns_VirtualFrameStatusFlg),
      | uint8(Ns_IncompleteFrameCntFlg),
      | uint8(Ns_OverflowCntFlg),
      | uint16(Ns_FrameBufferSize),
      | double(Ns_SampleTime)
      mask prompts: Ns_DeviceID "Device:"; Ns_ChannelNum "Channel number:"; Ns_FrameID "Frame ID:"; Ns_IsVirtualFrame "Belong to a virtual frame"; Ns_RoleInVirtualFrame "Position in virtual frame:"; Ns_HeaderFrameID "Header frame ID:"; Ns_VirtualFrameStatusFlg "Current virtural frame status output"; Ns_IncompleteFrameCntFlg "Incomplete virtual frame count output"; Ns_OverflowCntFlg "Overflow count output"; Ns_FrameBufferSize "Frame buffer size:"; Ns_SampleTime "Sample time:"
      mask init:
      | NSTC297CANReceive_callback('portlabels');
      mask TypeOptions Ns_DeviceID: General Control Unit Gen2 | ADAS Control Unit Gen2
      mask TypeOptions Ns_ChannelNum: 0 | 1 | 2 | 3 | 4 | 5
      mask Callback Ns_IsVirtualFrame: NSTC297CANReceive_callback('Belong to a virtual frame');
      mask TypeOptions Ns_RoleInVirtualFrame: Header Frame | Data Frame | Trailer Frame
      mask Callback Ns_RoleInVirtualFrame: NSTC297CANReceive_callback('Position in virtual frame');
      mask Display: color('blue');text(0.02,0.9,'NovSteeds TC297','horizontalAlignment','left');color('blue');text(0.5,0.7,'CAN Receive','horizontalAlignment','center');color('black');text(0.5,0.6,'Channel: 5','horizontalAlignment','center');text(0.5,0.5,'ID: 1824','horizontalAlignment','center');text(0.5,0.4,'Virtual Frame: No','horizontalAlignment','center');port_label('output',1, 'RemainderCnt');port_label('output',2, 'Msg');
  S-Function12 : S-Function  FunctionName=NSTC297CANReceiveBlkLib  Parameters=|  SFunctionDeploymentMode=off  EnableBusSupport=off  mask(NSTC297 CAN Receive){Ns_DeviceID=ADAS Control Unit Gen2, Ns_ChannelNum=5, Ns_FrameID=1828, Ns_IsVirtualFrame=off, Ns_RoleInVirtualFrame=Header Frame, Ns_HeaderFrameID=0, Ns_VirtualFrameStatusFlg=off, Ns_IncompleteFrameCntFlg=off, Ns_OverflowCntFlg=off, Ns_FrameBufferSize=1, Ns_SampleTime=0.05}
      | uint16(Ns_DeviceID),
      | uint16(Ns_ChannelNum),
      | uint32(Ns_FrameID),
      | uint8(Ns_IsVirtualFrame),
      | uint16(Ns_RoleInVirtualFrame),
      | uint32(Ns_HeaderFrameID),
      | uint8(Ns_VirtualFrameStatusFlg),
      | uint8(Ns_IncompleteFrameCntFlg),
      | uint8(Ns_OverflowCntFlg),
      | uint16(Ns_FrameBufferSize),
      | double(Ns_SampleTime)
      mask prompts: Ns_DeviceID "Device:"; Ns_ChannelNum "Channel number:"; Ns_FrameID "Frame ID:"; Ns_IsVirtualFrame "Belong to a virtual frame"; Ns_RoleInVirtualFrame "Position in virtual frame:"; Ns_HeaderFrameID "Header frame ID:"; Ns_VirtualFrameStatusFlg "Current virtural frame status output"; Ns_IncompleteFrameCntFlg "Incomplete virtual frame count output"; Ns_OverflowCntFlg "Overflow count output"; Ns_FrameBufferSize "Frame buffer size:"; Ns_SampleTime "Sample time:"
      mask init:
      | NSTC297CANReceive_callback('portlabels');
      mask TypeOptions Ns_DeviceID: General Control Unit Gen2 | ADAS Control Unit Gen2
      mask TypeOptions Ns_ChannelNum: 0 | 1 | 2 | 3 | 4 | 5
      mask Callback Ns_IsVirtualFrame: NSTC297CANReceive_callback('Belong to a virtual frame');
      mask TypeOptions Ns_RoleInVirtualFrame: Header Frame | Data Frame | Trailer Frame
      mask Callback Ns_RoleInVirtualFrame: NSTC297CANReceive_callback('Position in virtual frame');
      mask Display: color('blue');text(0.02,0.9,'NovSteeds TC297','horizontalAlignment','left');color('blue');text(0.5,0.7,'CAN Receive','horizontalAlignment','center');color('black');text(0.5,0.6,'Channel: 5','horizontalAlignment','center');text(0.5,0.5,'ID: 1828','horizontalAlignment','center');text(0.5,0.4,'Virtual Frame: No','horizontalAlignment','center');port_label('output',1, 'RemainderCnt');port_label('output',2, 'Msg');
  S-Function13 : S-Function  FunctionName=NSTC297CANReceiveBlkLib  Parameters=|  SFunctionDeploymentMode=off  EnableBusSupport=off  mask(NSTC297 CAN Receive){Ns_DeviceID=ADAS Control Unit Gen2, Ns_ChannelNum=5, Ns_FrameID=1832, Ns_IsVirtualFrame=off, Ns_RoleInVirtualFrame=Header Frame, Ns_HeaderFrameID=0, Ns_VirtualFrameStatusFlg=off, Ns_IncompleteFrameCntFlg=off, Ns_OverflowCntFlg=off, Ns_FrameBufferSize=1, Ns_SampleTime=0.05}
      | uint16(Ns_DeviceID),
      | uint16(Ns_ChannelNum),
      | uint32(Ns_FrameID),
      | uint8(Ns_IsVirtualFrame),
      | uint16(Ns_RoleInVirtualFrame),
      | uint32(Ns_HeaderFrameID),
      | uint8(Ns_VirtualFrameStatusFlg),
      | uint8(Ns_IncompleteFrameCntFlg),
      | uint8(Ns_OverflowCntFlg),
      | uint16(Ns_FrameBufferSize),
      | double(Ns_SampleTime)
      mask prompts: Ns_DeviceID "Device:"; Ns_ChannelNum "Channel number:"; Ns_FrameID "Frame ID:"; Ns_IsVirtualFrame "Belong to a virtual frame"; Ns_RoleInVirtualFrame "Position in virtual frame:"; Ns_HeaderFrameID "Header frame ID:"; Ns_VirtualFrameStatusFlg "Current virtural frame status output"; Ns_IncompleteFrameCntFlg "Incomplete virtual frame count output"; Ns_OverflowCntFlg "Overflow count output"; Ns_FrameBufferSize "Frame buffer size:"; Ns_SampleTime "Sample time:"
      mask init:
      | NSTC297CANReceive_callback('portlabels');
      mask TypeOptions Ns_DeviceID: General Control Unit Gen2 | ADAS Control Unit Gen2
      mask TypeOptions Ns_ChannelNum: 0 | 1 | 2 | 3 | 4 | 5
      mask Callback Ns_IsVirtualFrame: NSTC297CANReceive_callback('Belong to a virtual frame');
      mask TypeOptions Ns_RoleInVirtualFrame: Header Frame | Data Frame | Trailer Frame
      mask Callback Ns_RoleInVirtualFrame: NSTC297CANReceive_callback('Position in virtual frame');
      mask Display: color('blue');text(0.02,0.9,'NovSteeds TC297','horizontalAlignment','left');color('blue');text(0.5,0.7,'CAN Receive','horizontalAlignment','center');color('black');text(0.5,0.6,'Channel: 5','horizontalAlignment','center');text(0.5,0.5,'ID: 1832','horizontalAlignment','center');text(0.5,0.4,'Virtual Frame: No','horizontalAlignment','center');port_label('output',1, 'RemainderCnt');port_label('output',2, 'Msg');
  S-Function14 : S-Function  FunctionName=NSTC297CANReceiveBlkLib  Parameters=|  SFunctionDeploymentMode=off  EnableBusSupport=off  mask(NSTC297 CAN Receive){Ns_DeviceID=ADAS Control Unit Gen2, Ns_ChannelNum=5, Ns_FrameID=1836, Ns_IsVirtualFrame=off, Ns_RoleInVirtualFrame=Header Frame, Ns_HeaderFrameID=0, Ns_VirtualFrameStatusFlg=off, Ns_IncompleteFrameCntFlg=off, Ns_OverflowCntFlg=off, Ns_FrameBufferSize=1, Ns_SampleTime=0.05}
      | uint16(Ns_DeviceID),
      | uint16(Ns_ChannelNum),
      | uint32(Ns_FrameID),
      | uint8(Ns_IsVirtualFrame),
      | uint16(Ns_RoleInVirtualFrame),
      | uint32(Ns_HeaderFrameID),
      | uint8(Ns_VirtualFrameStatusFlg),
      | uint8(Ns_IncompleteFrameCntFlg),
      | uint8(Ns_OverflowCntFlg),
      | uint16(Ns_FrameBufferSize),
      | double(Ns_SampleTime)
      mask prompts: Ns_DeviceID "Device:"; Ns_ChannelNum "Channel number:"; Ns_FrameID "Frame ID:"; Ns_IsVirtualFrame "Belong to a virtual frame"; Ns_RoleInVirtualFrame "Position in virtual frame:"; Ns_HeaderFrameID "Header frame ID:"; Ns_VirtualFrameStatusFlg "Current virtural frame status output"; Ns_IncompleteFrameCntFlg "Incomplete virtual frame count output"; Ns_OverflowCntFlg "Overflow count output"; Ns_FrameBufferSize "Frame buffer size:"; Ns_SampleTime "Sample time:"
      mask init:
      | NSTC297CANReceive_callback('portlabels');
      mask TypeOptions Ns_DeviceID: General Control Unit Gen2 | ADAS Control Unit Gen2
      mask TypeOptions Ns_ChannelNum: 0 | 1 | 2 | 3 | 4 | 5
      mask Callback Ns_IsVirtualFrame: NSTC297CANReceive_callback('Belong to a virtual frame');
      mask TypeOptions Ns_RoleInVirtualFrame: Header Frame | Data Frame | Trailer Frame
      mask Callback Ns_RoleInVirtualFrame: NSTC297CANReceive_callback('Position in virtual frame');
      mask Display: color('blue');text(0.02,0.9,'NovSteeds TC297','horizontalAlignment','left');color('blue');text(0.5,0.7,'CAN Receive','horizontalAlignment','center');color('black');text(0.5,0.6,'Channel: 5','horizontalAlignment','center');text(0.5,0.5,'ID: 1836','horizontalAlignment','center');text(0.5,0.4,'Virtual Frame: No','horizontalAlignment','center');port_label('output',1, 'RemainderCnt');port_label('output',2, 'Msg');
  S-Function2 : S-Function  FunctionName=NSTC297CANReceiveBlkLib  Parameters=|  SFunctionDeploymentMode=off  EnableBusSupport=off  mask(NSTC297 CAN Receive){Ns_DeviceID=ADAS Control Unit Gen2, Ns_ChannelNum=5, Ns_FrameID=1800, Ns_IsVirtualFrame=off, Ns_RoleInVirtualFrame=Header Frame, Ns_HeaderFrameID=0, Ns_VirtualFrameStatusFlg=off, Ns_IncompleteFrameCntFlg=off, Ns_OverflowCntFlg=off, Ns_FrameBufferSize=1, Ns_SampleTime=0.05}
      | uint16(Ns_DeviceID),
      | uint16(Ns_ChannelNum),
      | uint32(Ns_FrameID),
      | uint8(Ns_IsVirtualFrame),
      | uint16(Ns_RoleInVirtualFrame),
      | uint32(Ns_HeaderFrameID),
      | uint8(Ns_VirtualFrameStatusFlg),
      | uint8(Ns_IncompleteFrameCntFlg),
      | uint8(Ns_OverflowCntFlg),
      | uint16(Ns_FrameBufferSize),
      | double(Ns_SampleTime)
      mask prompts: Ns_DeviceID "Device:"; Ns_ChannelNum "Channel number:"; Ns_FrameID "Frame ID:"; Ns_IsVirtualFrame "Belong to a virtual frame"; Ns_RoleInVirtualFrame "Position in virtual frame:"; Ns_HeaderFrameID "Header frame ID:"; Ns_VirtualFrameStatusFlg "Current virtural frame status output"; Ns_IncompleteFrameCntFlg "Incomplete virtual frame count output"; Ns_OverflowCntFlg "Overflow count output"; Ns_FrameBufferSize "Frame buffer size:"; Ns_SampleTime "Sample time:"
      mask init:
      | NSTC297CANReceive_callback('portlabels');
      mask TypeOptions Ns_DeviceID: General Control Unit Gen2 | ADAS Control Unit Gen2
      mask TypeOptions Ns_ChannelNum: 0 | 1 | 2 | 3 | 4 | 5
      mask Callback Ns_IsVirtualFrame: NSTC297CANReceive_callback('Belong to a virtual frame');
      mask TypeOptions Ns_RoleInVirtualFrame: Header Frame | Data Frame | Trailer Frame
      mask Callback Ns_RoleInVirtualFrame: NSTC297CANReceive_callback('Position in virtual frame');
      mask Display: color('blue');text(0.02,0.9,'NovSteeds TC297','horizontalAlignment','left');color('blue');text(0.5,0.7,'CAN Receive','horizontalAlignment','center');color('black');text(0.5,0.6,'Channel: 5','horizontalAlignment','center');text(0.5,0.5,'ID: 1800','horizontalAlignment','center');text(0.5,0.4,'Virtual Frame: No','horizontalAlignment','center');port_label('output',1, 'RemainderCnt');port_label('output',2, 'Msg');
  S-Function3 : S-Function  FunctionName=NSTC297CANReceiveBlkLib  Parameters=|  SFunctionDeploymentMode=off  EnableBusSupport=off  mask(NSTC297 CAN Receive){Ns_DeviceID=ADAS Control Unit Gen2, Ns_ChannelNum=5, Ns_FrameID=1804, Ns_IsVirtualFrame=off, Ns_RoleInVirtualFrame=Header Frame, Ns_HeaderFrameID=0, Ns_VirtualFrameStatusFlg=off, Ns_IncompleteFrameCntFlg=off, Ns_OverflowCntFlg=off, Ns_FrameBufferSize=1, Ns_SampleTime=0.05}
      | uint16(Ns_DeviceID),
      | uint16(Ns_ChannelNum),
      | uint32(Ns_FrameID),
      | uint8(Ns_IsVirtualFrame),
      | uint16(Ns_RoleInVirtualFrame),
      | uint32(Ns_HeaderFrameID),
      | uint8(Ns_VirtualFrameStatusFlg),
      | uint8(Ns_IncompleteFrameCntFlg),
      | uint8(Ns_OverflowCntFlg),
      | uint16(Ns_FrameBufferSize),
      | double(Ns_SampleTime)
      mask prompts: Ns_DeviceID "Device:"; Ns_ChannelNum "Channel number:"; Ns_FrameID "Frame ID:"; Ns_IsVirtualFrame "Belong to a virtual frame"; Ns_RoleInVirtualFrame "Position in virtual frame:"; Ns_HeaderFrameID "Header frame ID:"; Ns_VirtualFrameStatusFlg "Current virtural frame status output"; Ns_IncompleteFrameCntFlg "Incomplete virtual frame count output"; Ns_OverflowCntFlg "Overflow count output"; Ns_FrameBufferSize "Frame buffer size:"; Ns_SampleTime "Sample time:"
      mask init:
      | NSTC297CANReceive_callback('portlabels');
      mask TypeOptions Ns_DeviceID: General Control Unit Gen2 | ADAS Control Unit Gen2
      mask TypeOptions Ns_ChannelNum: 0 | 1 | 2 | 3 | 4 | 5
      mask Callback Ns_IsVirtualFrame: NSTC297CANReceive_callback('Belong to a virtual frame');
      mask TypeOptions Ns_RoleInVirtualFrame: Header Frame | Data Frame | Trailer Frame
      mask Callback Ns_RoleInVirtualFrame: NSTC297CANReceive_callback('Position in virtual frame');
      mask Display: color('blue');text(0.02,0.9,'NovSteeds TC297','horizontalAlignment','left');color('blue');text(0.5,0.7,'CAN Receive','horizontalAlignment','center');color('black');text(0.5,0.6,'Channel: 5','horizontalAlignment','center');text(0.5,0.5,'ID: 1804','horizontalAlignment','center');text(0.5,0.4,'Virtual Frame: No','horizontalAlignment','center');port_label('output',1, 'RemainderCnt');port_label('output',2, 'Msg');
  S-Function4 : S-Function  FunctionName=NSTC297CANReceiveBlkLib  Parameters=|  SFunctionDeploymentMode=off  EnableBusSupport=off  mask(NSTC297 CAN Receive){Ns_DeviceID=ADAS Control Unit Gen2, Ns_ChannelNum=5, Ns_FrameID=1808, Ns_IsVirtualFrame=off, Ns_RoleInVirtualFrame=Header Frame, Ns_HeaderFrameID=0, Ns_VirtualFrameStatusFlg=off, Ns_IncompleteFrameCntFlg=off, Ns_OverflowCntFlg=off, Ns_FrameBufferSize=1, Ns_SampleTime=0.05}
      | uint16(Ns_DeviceID),
      | uint16(Ns_ChannelNum),
      | uint32(Ns_FrameID),
      | uint8(Ns_IsVirtualFrame),
      | uint16(Ns_RoleInVirtualFrame),
      | uint32(Ns_HeaderFrameID),
      | uint8(Ns_VirtualFrameStatusFlg),
      | uint8(Ns_IncompleteFrameCntFlg),
      | uint8(Ns_OverflowCntFlg),
      | uint16(Ns_FrameBufferSize),
      | double(Ns_SampleTime)
      mask prompts: Ns_DeviceID "Device:"; Ns_ChannelNum "Channel number:"; Ns_FrameID "Frame ID:"; Ns_IsVirtualFrame "Belong to a virtual frame"; Ns_RoleInVirtualFrame "Position in virtual frame:"; Ns_HeaderFrameID "Header frame ID:"; Ns_VirtualFrameStatusFlg "Current virtural frame status output"; Ns_IncompleteFrameCntFlg "Incomplete virtual frame count output"; Ns_OverflowCntFlg "Overflow count output"; Ns_FrameBufferSize "Frame buffer size:"; Ns_SampleTime "Sample time:"
      mask init:
      | NSTC297CANReceive_callback('portlabels');
      mask TypeOptions Ns_DeviceID: General Control Unit Gen2 | ADAS Control Unit Gen2
      mask TypeOptions Ns_ChannelNum: 0 | 1 | 2 | 3 | 4 | 5
      mask Callback Ns_IsVirtualFrame: NSTC297CANReceive_callback('Belong to a virtual frame');
      mask TypeOptions Ns_RoleInVirtualFrame: Header Frame | Data Frame | Trailer Frame
      mask Callback Ns_RoleInVirtualFrame: NSTC297CANReceive_callback('Position in virtual frame');
      mask Display: color('blue');text(0.02,0.9,'NovSteeds TC297','horizontalAlignment','left');color('blue');text(0.5,0.7,'CAN Receive','horizontalAlignment','center');color('black');text(0.5,0.6,'Channel: 5','horizontalAlignment','center');text(0.5,0.5,'ID: 1808','horizontalAlignment','center');text(0.5,0.4,'Virtual Frame: No','horizontalAlignment','center');port_label('output',1, 'RemainderCnt');port_label('output',2, 'Msg');
  S-Function5 : S-Function  FunctionName=NSTC297CANReceiveBlkLib  Parameters=|  SFunctionDeploymentMode=off  EnableBusSupport=off  mask(NSTC297 CAN Receive){Ns_DeviceID=ADAS Control Unit Gen2, Ns_ChannelNum=5, Ns_FrameID=1812, Ns_IsVirtualFrame=off, Ns_RoleInVirtualFrame=Header Frame, Ns_HeaderFrameID=0, Ns_VirtualFrameStatusFlg=off, Ns_IncompleteFrameCntFlg=off, Ns_OverflowCntFlg=off, Ns_FrameBufferSize=1, Ns_SampleTime=0.05}
      | uint16(Ns_DeviceID),
      | uint16(Ns_ChannelNum),
      | uint32(Ns_FrameID),
      | uint8(Ns_IsVirtualFrame),
      | uint16(Ns_RoleInVirtualFrame),
      | uint32(Ns_HeaderFrameID),
      | uint8(Ns_VirtualFrameStatusFlg),
      | uint8(Ns_IncompleteFrameCntFlg),
      | uint8(Ns_OverflowCntFlg),
      | uint16(Ns_FrameBufferSize),
      | double(Ns_SampleTime)
      mask prompts: Ns_DeviceID "Device:"; Ns_ChannelNum "Channel number:"; Ns_FrameID "Frame ID:"; Ns_IsVirtualFrame "Belong to a virtual frame"; Ns_RoleInVirtualFrame "Position in virtual frame:"; Ns_HeaderFrameID "Header frame ID:"; Ns_VirtualFrameStatusFlg "Current virtural frame status output"; Ns_IncompleteFrameCntFlg "Incomplete virtual frame count output"; Ns_OverflowCntFlg "Overflow count output"; Ns_FrameBufferSize "Frame buffer size:"; Ns_SampleTime "Sample time:"
      mask init:
      | NSTC297CANReceive_callback('portlabels');
      mask TypeOptions Ns_DeviceID: General Control Unit Gen2 | ADAS Control Unit Gen2
      mask TypeOptions Ns_ChannelNum: 0 | 1 | 2 | 3 | 4 | 5
      mask Callback Ns_IsVirtualFrame: NSTC297CANReceive_callback('Belong to a virtual frame');
      mask TypeOptions Ns_RoleInVirtualFrame: Header Frame | Data Frame | Trailer Frame
      mask Callback Ns_RoleInVirtualFrame: NSTC297CANReceive_callback('Position in virtual frame');
      mask Display: color('blue');text(0.02,0.9,'NovSteeds TC297','horizontalAlignment','left');color('blue');text(0.5,0.7,'CAN Receive','horizontalAlignment','center');color('black');text(0.5,0.6,'Channel: 5','horizontalAlignment','center');text(0.5,0.5,'ID: 1812','horizontalAlignment','center');text(0.5,0.4,'Virtual Frame: No','horizontalAlignment','center');port_label('output',1, 'RemainderCnt');port_label('output',2, 'Msg');
  S-Function6 : S-Function  FunctionName=NSTC297CANReceiveBlkLib  Parameters=|  SFunctionDeploymentMode=off  EnableBusSupport=off  mask(NSTC297 CAN Receive){Ns_DeviceID=ADAS Control Unit Gen2, Ns_ChannelNum=5, Ns_FrameID=1792, Ns_IsVirtualFrame=off, Ns_RoleInVirtualFrame=Header Frame, Ns_HeaderFrameID=0, Ns_VirtualFrameStatusFlg=off, Ns_IncompleteFrameCntFlg=off, Ns_OverflowCntFlg=off, Ns_FrameBufferSize=1, Ns_SampleTime=0.05}
      | uint16(Ns_DeviceID),
      | uint16(Ns_ChannelNum),
      | uint32(Ns_FrameID),
      | uint8(Ns_IsVirtualFrame),
      | uint16(Ns_RoleInVirtualFrame),
      | uint32(Ns_HeaderFrameID),
      | uint8(Ns_VirtualFrameStatusFlg),
      | uint8(Ns_IncompleteFrameCntFlg),
      | uint8(Ns_OverflowCntFlg),
      | uint16(Ns_FrameBufferSize),
      | double(Ns_SampleTime)
      mask prompts: Ns_DeviceID "Device:"; Ns_ChannelNum "Channel number:"; Ns_FrameID "Frame ID:"; Ns_IsVirtualFrame "Belong to a virtual frame"; Ns_RoleInVirtualFrame "Position in virtual frame:"; Ns_HeaderFrameID "Header frame ID:"; Ns_VirtualFrameStatusFlg "Current virtural frame status output"; Ns_IncompleteFrameCntFlg "Incomplete virtual frame count output"; Ns_OverflowCntFlg "Overflow count output"; Ns_FrameBufferSize "Frame buffer size:"; Ns_SampleTime "Sample time:"
      mask init:
      | NSTC297CANReceive_callback('portlabels');
      mask TypeOptions Ns_DeviceID: General Control Unit Gen2 | ADAS Control Unit Gen2
      mask TypeOptions Ns_ChannelNum: 0 | 1 | 2 | 3 | 4 | 5
      mask Callback Ns_IsVirtualFrame: NSTC297CANReceive_callback('Belong to a virtual frame');
      mask TypeOptions Ns_RoleInVirtualFrame: Header Frame | Data Frame | Trailer Frame
      mask Callback Ns_RoleInVirtualFrame: NSTC297CANReceive_callback('Position in virtual frame');
      mask Display: color('blue');text(0.02,0.9,'NovSteeds TC297','horizontalAlignment','left');color('blue');text(0.5,0.7,'CAN Receive','horizontalAlignment','center');color('black');text(0.5,0.6,'Channel: 5','horizontalAlignment','center');text(0.5,0.5,'ID: 1792','horizontalAlignment','center');text(0.5,0.4,'Virtual Frame: No','horizontalAlignment','center');port_label('output',1, 'RemainderCnt');port_label('output',2, 'Msg');
  S-Function9 : S-Function  FunctionName=NSTC297CANReceiveBlkLib  Parameters=|  SFunctionDeploymentMode=off  EnableBusSupport=off  mask(NSTC297 CAN Receive){Ns_DeviceID=ADAS Control Unit Gen2, Ns_ChannelNum=5, Ns_FrameID=1816, Ns_IsVirtualFrame=off, Ns_RoleInVirtualFrame=Header Frame, Ns_HeaderFrameID=0, Ns_VirtualFrameStatusFlg=off, Ns_IncompleteFrameCntFlg=off, Ns_OverflowCntFlg=off, Ns_FrameBufferSize=1, Ns_SampleTime=0.05}
      | uint16(Ns_DeviceID),
      | uint16(Ns_ChannelNum),
      | uint32(Ns_FrameID),
      | uint8(Ns_IsVirtualFrame),
      | uint16(Ns_RoleInVirtualFrame),
      | uint32(Ns_HeaderFrameID),
      | uint8(Ns_VirtualFrameStatusFlg),
      | uint8(Ns_IncompleteFrameCntFlg),
      | uint8(Ns_OverflowCntFlg),
      | uint16(Ns_FrameBufferSize),
      | double(Ns_SampleTime)
      mask prompts: Ns_DeviceID "Device:"; Ns_ChannelNum "Channel number:"; Ns_FrameID "Frame ID:"; Ns_IsVirtualFrame "Belong to a virtual frame"; Ns_RoleInVirtualFrame "Position in virtual frame:"; Ns_HeaderFrameID "Header frame ID:"; Ns_VirtualFrameStatusFlg "Current virtural frame status output"; Ns_IncompleteFrameCntFlg "Incomplete virtual frame count output"; Ns_OverflowCntFlg "Overflow count output"; Ns_FrameBufferSize "Frame buffer size:"; Ns_SampleTime "Sample time:"
      mask init:
      | NSTC297CANReceive_callback('portlabels');
      mask TypeOptions Ns_DeviceID: General Control Unit Gen2 | ADAS Control Unit Gen2
      mask TypeOptions Ns_ChannelNum: 0 | 1 | 2 | 3 | 4 | 5
      mask Callback Ns_IsVirtualFrame: NSTC297CANReceive_callback('Belong to a virtual frame');
      mask TypeOptions Ns_RoleInVirtualFrame: Header Frame | Data Frame | Trailer Frame
      mask Callback Ns_RoleInVirtualFrame: NSTC297CANReceive_callback('Position in virtual frame');
      mask Display: color('blue');text(0.02,0.9,'NovSteeds TC297','horizontalAlignment','left');color('blue');text(0.5,0.7,'CAN Receive','horizontalAlignment','center');color('black');text(0.5,0.6,'Channel: 5','horizontalAlignment','center');text(0.5,0.5,'ID: 1816','horizontalAlignment','center');text(0.5,0.4,'Virtual Frame: No','horizontalAlignment','center');port_label('output',1, 'RemainderCnt');port_label('output',2, 'Msg');
  CmrObjRx_bsObjInfo : Outport
  tag scope: Id0=global, Id10=global, Id11=global, Id1=global, Id2=global, Id3=global, Id4=global, Id5=global, Id6=global, Id7=global, Id8=global, Id9=global
  wires:
  CAN Unpack7/4 -> Data Type Conversion3/1
  CAN Unpack1/6 -> Data Type Conversion13/1
  CAN Unpack4/4 -> Data Type Conversion32/1
  CAN Unpack3/6 -> Data Type Conversion27/1
  CAN Unpack1/4 -> Data Type Conversion11/1
  CAN Unpack3/2 -> Data Type Conversion23/1
  CAN Unpack3/7 -> Data Type Conversion28/1
  CAN Unpack1/1 -> Data Type Conversion8/1
  CAN Unpack4/3 -> Data Type Conversion31/1
  CAN Unpack5/7 -> Data Type Conversion42/1
  CAN Unpack7/6 -> Data Type Conversion6/1
  CAN Unpack7/7 -> Data Type Conversion7/1
  CAN Unpack4/6 -> Data Type Conversion34/1
  CAN Unpack3/5 -> Data Type Conversion26/1
  CAN Unpack3/4 -> Data Type Conversion25/1
  Data Type Conversion38/1 -> Bus Creator17/3  "Left_Angle"
  Data Type Conversion30/1 -> [Id4], Bus Creator16/2  "Identifier"
  Data Type Conversion35/1 -> Bus Creator16/7  "Right_Angle"
  Data Type Conversion29/1 -> Bus Creator16/1  "Class"
  Data Type Conversion8/1 -> Bus Creator13/1  "Class"
  CAN Unpack2/7 -> Data Type Conversion21/1
  CAN Unpack7/1 -> Data Type Conversion4/1
  Data Type Conversion25/1 -> Bus Creator15/4  "Longitudinal_Distance"
  Data Type Conversion36/1 -> Bus Creator17/1  "Class"
  Data Type Conversion21/1 -> Bus Creator14/7  "Right_Angle"
  CAN Unpack5/1 -> Data Type Conversion36/1
  Data Type Conversion33/1 -> Bus Creator16/5  "Message_Counter"
  Data Type Conversion20/1 -> Bus Creator14/6  "Relative_Velocity"
  Data Type Conversion3/1 -> Bus Creator/4  "Longitudinal_Distance"
  CAN Unpack7/5 -> Data Type Conversion5/1
  Bus Creator14/1 -> Bus Creator18/3  "vedio_obj_2"
  CAN Unpack7/3 -> Data Type Conversion2/1
  Data Type Conversion39/1 -> Bus Creator17/4  "Longitudinal_Distance"
  CAN Unpack4/2 -> Data Type Conversion30/1
  CAN Unpack1/5 -> Data Type Conversion12/1
  CAN Unpack7/2 -> Data Type Conversion1/1
  CAN Unpack5/3 -> Data Type Conversion38/1
  CAN Unpack1/3 -> Data Type Conversion10/1
  Data Type Conversion40/1 -> Bus Creator17/5  "Message_Counter"
  CAN Unpack5/5 -> Data Type Conversion40/1
  Data Type Conversion10/1 -> Bus Creator13/3  "Left_Angle"
  Data Type Conversion6/1 -> Bus Creator/6  "Relative_Velocity"
  Data Type Conversion22/1 -> Bus Creator15/1  "Class"
  Data Type Conversion5/1 -> Bus Creator/5  "Message_Counter"
  Data Type Conversion12/1 -> Bus Creator13/5  "Message_Counter"
  Bus Creator17/1 -> Bus Creator18/6  "vedio_obj_5"
  Data Type Conversion9/1 -> [Id1], Bus Creator13/2  "Identifier"
  CAN Unpack3/3 -> Data Type Conversion24/1
  Data Type Conversion26/1 -> Bus Creator15/5  "Message_Counter"
  Bus Creator/1 -> Bus Creator18/1  "vedio_obj_0"
  CAN Unpack5/6 -> Data Type Conversion41/1
  Data Type Conversion4/1 -> Bus Creator/1  "Class"
  Data Type Conversion18/1 -> Bus Creator14/4  "Longitudinal_Distance"
  Data Type Conversion13/1 -> Bus Creator13/6  "Relative_Velocity"
  CAN Unpack2/1 -> Data Type Conversion15/1
  Data Type Conversion24/1 -> Bus Creator15/3  "Left_Angle"
  Data Type Conversion1/1 -> [Id0], Bus Creator/2  "Identifier"
  Data Type Conversion31/1 -> Bus Creator16/3  "Left_Angle"
  Data Type Conversion16/1 -> [Id2], Bus Creator14/2  "Identifier"
  Data Type Conversion2/1 -> Bus Creator/3  "Left_Angle"
  Data Type Conversion17/1 -> Bus Creator14/3  "Left_Angle"
  CAN Unpack2/2 -> Data Type Conversion16/1
  CAN Unpack5/2 -> Data Type Conversion37/1
  Bus Creator18/1 -> CmrObjRx_bsObjInfo/1
  CAN Unpack2/6 -> Data Type Conversion20/1
  Data Type Conversion34/1 -> Bus Creator16/6  "Relative_Velocity"
  CAN Unpack4/1 -> Data Type Conversion29/1
  CAN Unpack4/5 -> Data Type Conversion33/1
  Data Type Conversion32/1 -> Bus Creator16/4  "Longitudinal_Distance"
  Data Type Conversion15/1 -> Bus Creator14/1  "Class"
  CAN Unpack2/4 -> Data Type Conversion18/1
  Data Type Conversion42/1 -> Bus Creator17/7  "Right_Angle"
  Data Type Conversion11/1 -> Bus Creator13/4  "Longitudinal_Distance"
  CAN Unpack3/1 -> Data Type Conversion22/1
  Data Type Conversion19/1 -> Bus Creator14/5  "Message_Counter"
  CAN Unpack5/4 -> Data Type Conversion39/1
  CAN Unpack2/3 -> Data Type Conversion17/1
  Bus Creator13/1 -> Bus Creator18/2  "vedio_obj_1"
  Data Type Conversion14/1 -> Bus Creator13/7  "Right_Angle"
  CAN Unpack2/5 -> Data Type Conversion19/1
  Bus Creator15/1 -> Bus Creator18/4  "vedio_obj_3"
  Bus Creator16/1 -> Bus Creator18/5  "vedio_obj_4"
  Data Type Conversion28/1 -> Bus Creator15/7  "Right_Angle"
  CAN Unpack1/2 -> Data Type Conversion9/1
  Data Type Conversion37/1 -> [Id5], Bus Creator17/2  "Identifier"
  CAN Unpack1/7 -> Data Type Conversion14/1
  CAN Unpack4/7 -> Data Type Conversion35/1
  Data Type Conversion27/1 -> Bus Creator15/6  "Relative_Velocity"
  Data Type Conversion7/1 -> Bus Creator/7  "Right_Angle"
  Data Type Conversion23/1 -> [Id3], Bus Creator15/2  "Identifier"
  Data Type Conversion41/1 -> Bus Creator17/6  "Relative_Velocity"
  S-Function6/2 -> CAN Unpack7/1
  S-Function1/2 -> CAN Unpack1/1
  S-Function2/2 -> CAN Unpack2/1
  S-Function3/2 -> CAN Unpack3/1
  S-Function4/2 -> CAN Unpack4/1
  S-Function5/2 -> CAN Unpack5/1
  S-Function9/2 -> CAN Unpack6/1
  Data Type Conversion48/1 -> Bus Creator19/6  "Relative_Velocity"
  Data Type Conversion44/1 -> [Id6], Bus Creator19/2  "Identifier"
  CAN Unpack6/4 -> Data Type Conversion46/1
  Data Type Conversion49/1 -> Bus Creator19/7  "Right_Angle"
  CAN Unpack6/2 -> Data Type Conversion44/1
  CAN Unpack6/6 -> Data Type Conversion48/1
  Bus Creator19/1 -> Bus Creator18/7  "vedio_obj_6"
  CAN Unpack6/5 -> Data Type Conversion47/1
  Data Type Conversion47/1 -> Bus Creator19/5  "Message_Counter"
  CAN Unpack6/3 -> Data Type Conversion45/1
  Data Type Conversion46/1 -> Bus Creator19/4  "Longitudinal_Distance"
  CAN Unpack6/1 -> Data Type Conversion43/1
  Data Type Conversion43/1 -> Bus Creator19/1  "Class"
  Data Type Conversion45/1 -> Bus Creator19/3  "Left_Angle"
  CAN Unpack6/7 -> Data Type Conversion49/1
  CAN Unpack8/7 -> Data Type Conversion56/1
  Data Type Conversion52/1 -> Bus Creator20/3  "Left_Angle"
  Data Type Conversion50/1 -> Bus Creator20/1  "Class"
  CAN Unpack8/1 -> Data Type Conversion50/1
  Data Type Conversion53/1 -> Bus Creator20/4  "Longitudinal_Distance"
  CAN Unpack8/3 -> Data Type Conversion52/1
  Data Type Conversion54/1 -> Bus Creator20/5  "Message_Counter"
  CAN Unpack8/5 -> Data Type Conversion54/1
  Bus Creator20/1 -> Bus Creator18/8  "vedio_obj_7"
  CAN Unpack8/6 -> Data Type Conversion55/1
  CAN Unpack8/2 -> Data Type Conversion51/1
  Data Type Conversion56/1 -> Bus Creator20/7  "Right_Angle"
  CAN Unpack8/4 -> Data Type Conversion53/1
  Data Type Conversion51/1 -> Bus Creator20/2, [Id7]  "Identifier"
  Data Type Conversion55/1 -> Bus Creator20/6  "Relative_Velocity"
  S-Function10/2 -> CAN Unpack8/1
  S-Function11/2 -> CAN Unpack9/1
  Data Type Conversion62/1 -> Bus Creator21/6  "Relative_Velocity"
  Data Type Conversion58/1 -> [Id8], Bus Creator21/2  "Identifier"
  CAN Unpack9/4 -> Data Type Conversion60/1
  Data Type Conversion63/1 -> Bus Creator21/7  "Right_Angle"
  CAN Unpack9/2 -> Data Type Conversion58/1
  CAN Unpack9/6 -> Data Type Conversion62/1
  Bus Creator21/1 -> Bus Creator18/9  "vedio_obj_8"
  CAN Unpack9/5 -> Data Type Conversion61/1
  Data Type Conversion61/1 -> Bus Creator21/5  "Message_Counter"
  CAN Unpack9/3 -> Data Type Conversion59/1
  Data Type Conversion60/1 -> Bus Creator21/4  "Longitudinal_Distance"
  CAN Unpack9/1 -> Data Type Conversion57/1
  Data Type Conversion57/1 -> Bus Creator21/1  "Class"
  Data Type Conversion59/1 -> Bus Creator21/3  "Left_Angle"
  CAN Unpack9/7 -> Data Type Conversion63/1
  CAN Unpack10/7 -> Data Type Conversion70/1
  Data Type Conversion66/1 -> Bus Creator22/3  "Left_Angle"
  Data Type Conversion64/1 -> Bus Creator22/1  "Class"
  CAN Unpack10/1 -> Data Type Conversion64/1
  Data Type Conversion67/1 -> Bus Creator22/4  "Longitudinal_Distance"
  CAN Unpack10/3 -> Data Type Conversion66/1
  Data Type Conversion68/1 -> Bus Creator22/5  "Message_Counter"
  CAN Unpack10/5 -> Data Type Conversion68/1
  Bus Creator22/1 -> Bus Creator18/10  "vedio_obj_9"
  CAN Unpack10/6 -> Data Type Conversion69/1
  CAN Unpack10/2 -> Data Type Conversion65/1
  Data Type Conversion70/1 -> Bus Creator22/7  "Right_Angle"
  CAN Unpack10/4 -> Data Type Conversion67/1
  Data Type Conversion65/1 -> [Id9], Bus Creator22/2  "Identifier"
  Data Type Conversion69/1 -> Bus Creator22/6  "Relative_Velocity"
  S-Function12/2 -> CAN Unpack10/1
  S-Function13/2 -> CAN Unpack11/1
  Data Type Conversion76/1 -> Bus Creator23/6  "Relative_Velocity"
  Data Type Conversion72/1 -> [Id10], Bus Creator23/2  "Identifier"
  CAN Unpack11/4 -> Data Type Conversion74/1
  Data Type Conversion77/1 -> Bus Creator23/7  "Right_Angle"
  CAN Unpack11/2 -> Data Type Conversion72/1
  CAN Unpack11/6 -> Data Type Conversion76/1
  Bus Creator23/1 -> Bus Creator18/11  "vedio_obj_10"
  CAN Unpack11/5 -> Data Type Conversion75/1
  Data Type Conversion75/1 -> Bus Creator23/5  "Message_Counter"
  CAN Unpack11/3 -> Data Type Conversion73/1
  Data Type Conversion74/1 -> Bus Creator23/4  "Longitudinal_Distance"
  CAN Unpack11/1 -> Data Type Conversion71/1
  Data Type Conversion71/1 -> Bus Creator23/1  "Class"
  Data Type Conversion73/1 -> Bus Creator23/3  "Left_Angle"
  CAN Unpack11/7 -> Data Type Conversion77/1
  CAN Unpack12/7 -> Data Type Conversion84/1
  Data Type Conversion80/1 -> Bus Creator24/3  "Left_Angle"
  Data Type Conversion78/1 -> Bus Creator24/1  "Class"
  CAN Unpack12/1 -> Data Type Conversion78/1
  Data Type Conversion81/1 -> Bus Creator24/4  "Longitudinal_Distance"
  CAN Unpack12/3 -> Data Type Conversion80/1
  Data Type Conversion82/1 -> Bus Creator24/5  "Message_Counter"
  CAN Unpack12/5 -> Data Type Conversion82/1
  Bus Creator24/1 -> Bus Creator18/12  "vedio_obj_11"
  CAN Unpack12/6 -> Data Type Conversion83/1
  CAN Unpack12/2 -> Data Type Conversion79/1
  Data Type Conversion84/1 -> Bus Creator24/7  "Right_Angle"
  CAN Unpack12/4 -> Data Type Conversion81/1
  Data Type Conversion79/1 -> [Id11], Bus Creator24/2  "Identifier"
  Data Type Conversion83/1 -> Bus Creator24/6  "Relative_Velocity"
  S-Function14/2 -> CAN Unpack12/1
